simulink model "simulink3"  (R2018a)
settings: Solver=VariableStepAuto  StartTime=0.0  StopTime=10.0  RelTol=1e-3
settings Model: Creator=Surja Kamal Ghosh  LastModifiedBy=Surja Kamal Ghosh

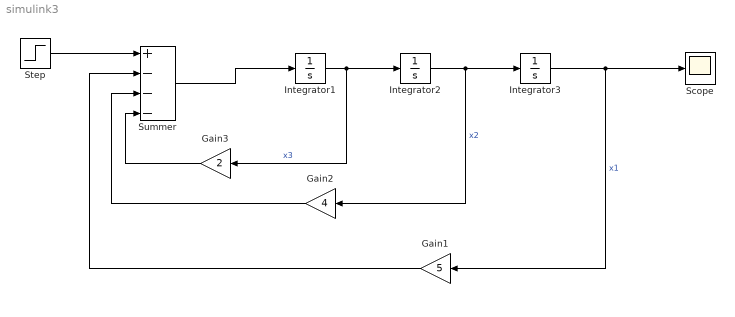
== system simulink3 ==
  Gain1 : Gain  Gain=5
  Gain2 : Gain  Gain=4
  Gain3 : Gain  Gain=2
  Integrator1 : Integrator
  Integrator2 : Integrator
  Integrator3 : Integrator
  Scope : Scope
  Step : Step  After=5  SampleTime=0
  Summer : Sum  Inputs=+---
  wires:
  Step/1 -> Summer/1
  Summer/1 -> Integrator1/1
  Integrator1/1 -> Integrator2/1, Gain3/1  "x3"
  Integrator2/1 -> Integrator3/1, Gain2/1  "x2"
  Integrator3/1 -> Gain1/1, Scope/1  "x1"
  Gain3/1 -> Summer/4
  Gain2/1 -> Summer/3
  Gain1/1 -> Summer/2
